simulink model "breaker_slower"  (R2023a)
settings: Solver=daessc  StartTime=0.0  StopTime=60*60*24  RelTol=1e-3
InitFcn:
  | to = 0.1;
  | V_G = 16.5e3;
  | V1 = 230e3;
  | V2 = 10.5e3;
  | V3 = 380;
  | 
  | P_G = 10e6;
  | S_T1 = 5e6;
  | S_T2 = S_T1;
undefined symbols (not defined in the file): A, B, C, D1, Dd, Delta, j
libraries: spsThreePhaseVIMeasurementLib x4, spsThreePhaseTransformerTwoWindingsLib x3, spsThreePhaseParallelRLCLoadLib x3, spsDistributedParametersLineLib x2, spsSeriesRLCBranchLib x2, spsControlledCurrentSourceLib x2, spsVoltageMeasurementLib x2, spsDieselMotorModel x1, spsExcitationSystemLib x1, spsPower3phPhasorLib x1, spsSynchronousMachinepuStandardLib x1, spsThreePhaseBreakerLib x1
settings Model: Creator=97033  LastModifiedBy=97033

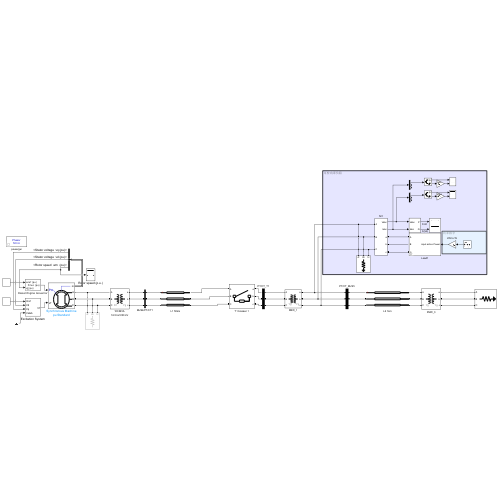
[thumbnail: Simulink's stored preview of the top-level diagram]
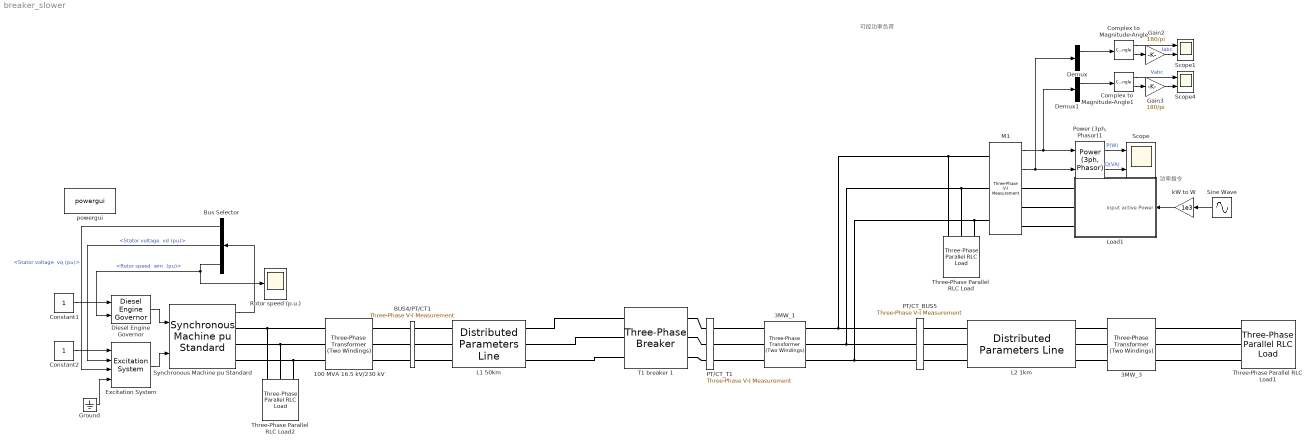
== system breaker_slower ==
  note: 功率指令
  note: 可控功率负荷
  100 MVA 16.5 kV/230 kV : spsThreePhaseTransformerTwoWindingsLib/Three-Phase Transformer (Two Windings)  Winding1Connection=Delta (D1)  Winding2Connection=Yg  CoreType=Three single-phase transformers  SetSaturation=off  Hysteresis=off  DataFile='hysteresis'  SetInitialFlux=off  Measurements=All measurements (V I Fluxes)  UNITS=pu  NominalPower=[P_G 50 ]  Winding1="[V_G 0.002  0.08]"  Winding2=[ V1 0.002 0.0576]  Rm=500  Lm=500  L0=0.5  Saturation="[ 0,0  ;  0.005,1.2  ;  1.0,1.4 ]"  InitialFluxes=[ 0.8 , -0.8 , 0.7 ]  BreakLoop=off  DiscreteSolver=Trapezoidal iterative  DataType=off  TransfoNumber=0
  3MW_1 : spsThreePhaseTransformerTwoWindingsLib/Three-Phase Transformer (Two Windings)  Winding1Connection=Yg  Winding2Connection=Yg  CoreType=Three single-phase transformers  SetSaturation=off  Hysteresis=off  DataFile='hysteresis'  SetInitialFlux=off  Measurements=None  UNITS=pu  NominalPower=[S_T1 , 50 ]  Winding1=[ V1 , 0.002 , 0.08 ]  Winding2=[ V2 , 0.002 , 0.08 ]  Rm=500  Lm=500  L0=0.5  Saturation=[ 0,0 ; 0.0024,1.2 ; 1.0,1.52 ]  InitialFluxes=[ 0.8 , -0.8 , 0.7 ]  BreakLoop=off  DiscreteSolver=Trapezoidal iterative  DataType=off  TransfoNumber=1
  3MW_3 : spsThreePhaseTransformerTwoWindingsLib/Three-Phase Transformer (Two Windings)  Winding1Connection=Yg  Winding2Connection=Yg  CoreType=Three single-phase transformers  SetSaturation=off  Hysteresis=off  DataFile='hysteresis'  SetInitialFlux=off  Measurements=None  UNITS=pu  NominalPower=[S_T1 , 50 ]  Winding1=[ V2 , 0.002 , 0.08 ]  Winding2=[ V3 , 0.002 , 0.08 ]  Rm=500  Lm=500  L0=0.5  Saturation=[ 0,0 ; 0.0024,1.2 ; 1.0,1.52 ]  InitialFluxes=[ 0.8 , -0.8 , 0.7 ]  BreakLoop=off  DiscreteSolver=Trapezoidal iterative  DataType=off  TransfoNumber=1
  BUS4/PT/CT1 : spsThreePhaseVIMeasurementLib/Three-Phase V-I Measurement  VoltageMeasurement=phase-to-ground  SetLabelV=on  LabelV=BUS4_Vabc  Vpu=off  VpuLL=off  CurrentMeasurement=yes  SetLabelI=on  LabelI=BUS4_Iabc  Ipu=off  Pbase=100e6  Vbase=500e3  OutputType=Complex  PhasorSimulation=on  PSBequivalent=0
  Bus Selector : BusSelector  OutputSignals="dq0 components.Stator voltage  vq (pu),dq0 components.Stator voltage  vd (pu),Mechanical.Rotor speed  wm  (pu)"
  Complex to Magnitude-Angle : ComplexToMagnitudeAngle
  Complex to Magnitude-Angle1 : ComplexToMagnitudeAngle
  Constant1 : Constant
  Constant2 : Constant
  Demux : Demux  Outputs=3
  Demux1 : Demux  Outputs=3
  Diesel Engine Governor : spsDieselMotorModel/Diesel Engine Governor  K=29  Tr=[0.01 0.02 0.2]  Ta=[0.25 0.009 0.0384]  Tlim=[0 1.1]  Td=0.024  Pm0=0.007343
  Excitation System : spsExcitationSystemLib/Excitation System  tr=20e-3  reg=[ 300, 0.001 ]  exc=[ 1, 0 ]  tgr=[ 0, 0 ]  damp=[ 0.001, 0.1 ]  sat=[ 0, 0 ]  lim=[ -11.5, 11.5, 0 ]  v0=[1 1.0072]
  Gain2 : Gain  Gain=180/pi
  Gain3 : Gain  Gain=180/pi
  Ground : Ground
  L1 50km : spsDistributedParametersLineLib/Distributed Parameters Line  Phases=3  Length=50  Frequency=50  Resistance="[0.1058  0.2758]"  Inductance="[2.3854e-3  3.220e-3]"  Capacitance="[17.65e-9  8.297e-9]"  x1=[8.11254497425638e-10 1435.76822832671 1413.84463935268;314.159265358979 314.159265358979 314.159265358979;-1.51704666570655 -1.26319034583497 -2.82717844992401]  x2=[7.80983845873745e-10 1443.20228947027 1421.37759574387;314.159265358979 314.159265358979 314.159265358979;-1.57738704185351 -1.26390237661045 -2.82798405384252]  x3=[3.89558894376792e-13 3.88420818677175 3.82284151982266;314.159265358979 314.159265358979 314.159265358979;-0.687252712637529 -1.36506185207182 -2.93068634651134]  x4=[2.29141256438702e-12 3.88291642642986 3.82686373555617;314.159265358979 314.159265358979 314.159265358979;-1.7204680603264 -1.26430606341361 -2.82682308359116]  x5=0.000324431464257091  V1=[1.093e-05 9.838e+04 9.838e+04;314.2 314.2 314.2;-0.3111 0.00854 -1.562]  V2=[1.093e-05 9.237e+04 9.237e+04;314.2 314.2 314.2;-0.3111 -0.2113 -1.782]  I1=[1.745e-08 2.849e+04 2.849e+04;314.2 314.2 314.2;-0.3423 2.9 1.329]  I2=[1.767e-08 2.9e+04 2.9e+04;314.2 314.2 314.2;-0.2816 -0.2391 -1.81]  nHarmo=1  Measurements=None  Decoupling=off  VsMag0=0  VrMag0=0  VsAngle0=0  VrAngle0=0  IsMag0=0  IrMag0=0  IsAngle0=0  IrAngle0=0
      settings: AttributesFormatString=\n
  L2 1km : spsDistributedParametersLineLib/Distributed Parameters Line  Phases=3  Length=1  Frequency=50  Resistance="[0.1058  0.2758]"  Inductance="[2.3854e-3  3.220e-3]"  Capacitance="[17.65e-9  8.297e-9]"  x1=[2.11924365740915e-09 78721.7359658811 223822.826299137;314.159265358979 314.159265358979 314.159265358979;-2.64962390305536 -0.00655028347033348 1.56395213727741]  x2=[2.12547837018316e-09 78715.0348375581 223803.77355008;314.159265358979 314.159265358979 314.159265358979;-2.64341726306893 -0.00667686374960178 1.56382555699814]  x3=[3.3655743288385e-11 199.928996109937 568.441135341219;314.159265358979 314.159265358979 314.159265358979;3.09267060703222 0.0270103950188096 1.59751281576664]  x4=[9.94540432532086e-12 228.454278999728 649.544649625245;314.159265358979 314.159265358979 314.159265358979;-1.5736701478916 -0.0379490943389389 1.53255332640882]  x5=6.48862928514182e-06  V1=[1.093e-05 9.838e+04 9.838e+04;314.2 314.2 314.2;-0.3111 0.00854 -1.562]  V2=[1.093e-05 9.237e+04 9.237e+04;314.2 314.2 314.2;-0.3111 -0.2113 -1.782]  I1=[1.745e-08 2.849e+04 2.849e+04;314.2 314.2 314.2;-0.3423 2.9 1.329]  I2=[1.767e-08 2.9e+04 2.9e+04;314.2 314.2 314.2;-0.2816 -0.2391 -1.81]  nHarmo=1  Measurements=None  Decoupling=off  VsMag0=0  VrMag0=0  VsAngle0=0  VrAngle0=0  IsMag0=0  IrMag0=0  IsAngle0=0  IrAngle0=0
      settings: AttributesFormatString=\n
  Load1 : Subsystem  mask{power_factor=1}
      mask DialogControl ParameterGroupVar Prompt: 参数
  M1 : spsThreePhaseVIMeasurementLib/Three-Phase V-I Measurement  VoltageMeasurement=phase-to-ground  SetLabelV=off  LabelV=V_Wind  Vpu=off  VpuLL=off  CurrentMeasurement=yes  SetLabelI=off  LabelI=I_Wind  Ipu=off  Pbase=6*1.5e6/0.9  Vbase=575  OutputType=Complex  PhasorSimulation=on  PSBequivalent=0
  PT/CT_BUS5 : spsThreePhaseVIMeasurementLib/Three-Phase V-I Measurement  VoltageMeasurement=phase-to-ground  SetLabelV=on  LabelV=BUS5_Vabc  Vpu=off  VpuLL=off  CurrentMeasurement=yes  SetLabelI=on  LabelI=BUS5_Iabc  Ipu=off  Pbase=6*1.5e6/0.9  Vbase=575  OutputType=Complex  PhasorSimulation=on  PSBequivalent=0
  PT/CT_T1 : spsThreePhaseVIMeasurementLib/Three-Phase V-I Measurement  VoltageMeasurement=phase-to-ground  SetLabelV=on  LabelV=V_T1  Vpu=off  VpuLL=off  CurrentMeasurement=yes  SetLabelI=on  LabelI=I_T1  Ipu=off  Pbase=6*1.5e6/0.9  Vbase=575  OutputType=Complex  PhasorSimulation=on  PSBequivalent=0
  "Power (3ph, Phasor)1" : spsPower3phPhasorLib/Power (3ph, Phasor)
  Rotor speed (p.u.) : Scope
  Scope : Scope  NumInputPorts=2
  Scope1 : Scope  NumInputPorts=2
  Scope4 : Scope  NumInputPorts=2
  Sine Wave : Sin  SineType=Sample based  Amplitude=5  Frequency=3600  SampleTime=60
  Synchronous Machine pu Standard : spsSynchronousMachinepuStandardLib/Synchronous Machine pu Standard  PresetModel=No  MechanicalLoad=Mechanical power Pm  ShowDetailedParameters=on  RotorType=Salient-pole  Units=per unit standard parameters  MeasurementBus=off  NominalParameters="[ P_G  V_G   50]"  Reactances1=[ 1.81, 0.3, 0.23, 1.76, 0.65, 0.25, 0.15 ]  Reactances2="[ 1.305, 0.296, 0.252, 0.474,  0.243,  0.18 ]"  dAxisTimeConstants=Open-circuit  qAxisTimeConstants=Short-circuit  TimeConstants1="[ 4.4849  0.0681  0.1  ]"  TimeConstants2=[ 8.0, 0.03, 1.0, 0.07 ]  TimeConstants3="[  4.49  0.0681  0.0513  ]"  TimeConstants4=[ 8.0, 0.03, 0.3371, 0.0295 ]  TimeConstants5=[ 1.01, 0.053, 0.1 ]  TimeConstants6=[ 1.3201, 0.023, 1.0, 0.07 ]  TimeConstants7=[0.012 0.003 0.003]  TimeConstants8=[ 1.3201, 0.0231, 0.3371, 0.0295 ]  StatorResistance=0.003  Mechanical=[3.7 0 1 ]  PolePairs=20  InitialConditions=[0 -89.802 0.00913935 0.00913935 0.00913935 -36.542 -156.542 83.458 1.00715]  SetSaturation=off  Saturation=[0.6404,0.7127,0.8441,0.9214,0.9956,1.082,1.19,1.316,1.457;0.7,0.7698,0.8872,0.9466,0.9969,1.046,1.1,1.151,1.201]  LoadFlowParameters=[1,0,0,0,0]  TsPowergui=0  TsBlock=-1  IterativeModel=Trapezoidal non iterative  IterativeDiscreteModel=Trapezoidal non iterative  BusType=swing  Pref=0  Qref=0  Qmin=-inf  Qmax=inf  PLF=0  QLF=0
  T1 breaker 1 : spsThreePhaseBreakerLib/Three-Phase Breaker  InitialState=open  SwitchA=on  SwitchB=on  SwitchC=on  SwitchTimes=0  External=off  BreakerResistance=1e-6  SnubberResistance=1e9  SnubberCapacitance=inf  Measurements=None
  Three-Phase Parallel RLC Load : spsThreePhaseParallelRLCLoadLib/Three-Phase Parallel RLC Load  LConnTagsString=A|B|C  Configuration=Y (grounded)  NominalVoltage=V2  Vabc=[1e3 1e3 1e3]  Vabcp=[1e3 1e3 1e3]  NominalFrequency=50  UnbalancedPower=off  ActivePower=1e6  InductivePower=0  CapacitivePower=0  Pabc=[10e3 9e3 11e3]  QLabc=[100 90 110]  QCabc=[100 90 110]  Pabcp=[10e3 9e3 11e3]  QLabcp=[100 90 110]  QCabcp=[100 90 110]  Measurements=None  LoadType=constant Z
  Three-Phase Parallel RLC Load1 : spsThreePhaseParallelRLCLoadLib/Three-Phase Parallel RLC Load  LConnTagsString=A|B|C  Configuration=Y (grounded)  NominalVoltage=V3  Vabc=[1e3 1e3 1e3]  Vabcp=[1e3 1e3 1e3]  NominalFrequency=50  UnbalancedPower=off  ActivePower=10e3  InductivePower=0  CapacitivePower=0  Pabc=[10e3 9e3 11e3]  QLabc=[100 90 110]  QCabc=[100 90 110]  Pabcp=[10e3 9e3 11e3]  QLabcp=[100 90 110]  QCabcp=[100 90 110]  Measurements=None  LoadType=constant Z
  Three-Phase Parallel RLC Load2 : spsThreePhaseParallelRLCLoadLib/Three-Phase Parallel RLC Load  LConnTagsString=A|B|C  Configuration=Y (floating)  NominalVoltage=V_G  Vabc=[1e3 1e3 1e3]  Vabcp=[1e3 1e3 1e3]  NominalFrequency=50  UnbalancedPower=off  ActivePower=1e3  InductivePower=0  CapacitivePower=0  Pabc=[10e3 9e3 11e3]  QLabc=[100 90 110]  QCabc=[100 90 110]  Pabcp=[10e3 9e3 11e3]  QLabcp=[100 90 110]  QCabcp=[100 90 110]  Measurements=None  LoadType=constant PQ
  kW to W : Gain  Gain=1e3
  powergui : sps_lib/powergui  Priority=1  SimulationMode=Phasor  SampleTime=50e-6  frequency=50  Iterations=50  frequencyindice=50  Pbase=100e6  ErrMax=1e-4  UnitsV=kV  UnitsW=MW  buscounter=0  FunctionMessages=off  echomessages=off  EnableUseOfTLC=off  CurrentSourceSwitches=off  DisableSnubberDevices=off  DisableRonSwitches=off  DisableVfSwitches=off  DisplayEquations=off  AutomaticDiscreteSolvers=off  SolverType=Tustin/Backward Euler (TBE)  Interpol=off  ExternalGateDelay=off  methode=off  Ts=100  x0status=blocks  SPID=on  SwTol=0  HookPort=off  NonlinearTolerance=1e-4  nMaxIteration=100  ContinueOnMaxIteration=off  RestoreLinks=warning  ResistiveCurrentMeasurement=off  Frange=[0:2:500]  Ylog=off  Xlog=on  ShowGrid=off  save=off  variable=ZData  structure=0  ZoomFFT=off  StartTime=0.0  cycles=1  DisplayStyle=1  fundamental=60  FreqAxis=off  MaxFrequency=1000  frequencyindicesteady=1  RmsSteady=1  display=off
  wires:
  Bus Selector/3 -> Diesel Engine Governor/2, Rotor speed (p.u.)/1  "<Rotor speed  wm  (pu)>"
  Ground/1 -> Excitation System/4
  Constant1/1 -> Diesel Engine Governor/1
  Bus Selector/1 -> Excitation System/3  "<Stator voltage  vq (pu)>"
  Constant2/1 -> Excitation System/1
  Diesel Engine Governor/1 -> Synchronous Machine pu Standard/1
  Bus Selector/2 -> Excitation System/2  "<Stator voltage  vd (pu)>"
  Excitation System/1 -> Synchronous Machine pu Standard/2
  Synchronous Machine pu Standard/1 -> Bus Selector/1
  Complex to Magnitude-Angle1/2 -> Gain3/1
  Complex to Magnitude-Angle1/1 -> Scope4/1  "Vabc"
  Complex to Magnitude-Angle/1 -> Scope1/1  "Iabc"
  Complex to Magnitude-Angle/2 -> Gain2/1
  Sine Wave/1 -> kW to W/1
  Demux1/1 -> Complex to Magnitude-Angle1/1
  Demux/1 -> Complex to Magnitude-Angle/1
  kW to W/1 -> Load1/1(input active Power)
  "Power (3ph, Phasor)1"/2 -> Scope/2  "Q(VA)"
  M1/2 -> Demux/1, "Power (3ph, Phasor)1"/2
  Gain3/1 -> Scope4/2
  Gain2/1 -> Scope1/2
  "Power (3ph, Phasor)1"/1 -> Scope/1  "P(W)"
  M1/1 -> Demux1/1, "Power (3ph, Phasor)1"/1
  connections:
  T1 breaker 1/LConn2 -- L1 50km/RConn2
  L1 50km/RConn1 -- T1 breaker 1/LConn1
  PT/CT_BUS5/RConn1 -- L2 1km/LConn1
  Three-Phase Parallel RLC Load2/LConn3 -- Synchronous Machine pu Standard/RConn3 -- 100 MVA 16.5 kV/230 kV/LConn3
  PT/CT_BUS5/RConn3 -- L2 1km/LConn3
  Synchronous Machine pu Standard/RConn2 -- Three-Phase Parallel RLC Load2/LConn2 -- 100 MVA 16.5 kV/230 kV/LConn2
  Three-Phase Parallel RLC Load/LConn1 -- 3MW_1/RConn1 -- PT/CT_BUS5/LConn1 -- M1/LConn1
  L1 50km/RConn3 -- T1 breaker 1/LConn3
  M1/LConn2 -- 3MW_1/RConn2 -- PT/CT_BUS5/LConn2 -- Three-Phase Parallel RLC Load/LConn2
  PT/CT_BUS5/RConn2 -- L2 1km/LConn2
  M1/LConn3 -- 3MW_1/RConn3 -- PT/CT_BUS5/LConn3 -- Three-Phase Parallel RLC Load/LConn3
  Synchronous Machine pu Standard/RConn1 -- Three-Phase Parallel RLC Load2/LConn1 -- 100 MVA 16.5 kV/230 kV/LConn1
  3MW_3/RConn2 -- Three-Phase Parallel RLC Load1/LConn2
  PT/CT_T1/RConn1 -- 3MW_1/LConn1
  3MW_3/LConn3 -- L2 1km/RConn3
  3MW_3/LConn1 -- L2 1km/RConn1
  L1 50km/LConn2 -- BUS4/PT/CT1/RConn2
  BUS4/PT/CT1/LConn2 -- 100 MVA 16.5 kV/230 kV/RConn2
  L1 50km/LConn3 -- BUS4/PT/CT1/RConn3
  PT/CT_T1/RConn2 -- 3MW_1/LConn2
  L1 50km/LConn1 -- BUS4/PT/CT1/RConn1
  Three-Phase Parallel RLC Load1/LConn1 -- 3MW_3/RConn1
  BUS4/PT/CT1/LConn1 -- 100 MVA 16.5 kV/230 kV/RConn1
  T1 breaker 1/RConn3 -- PT/CT_T1/LConn3
  3MW_3/LConn2 -- L2 1km/RConn2
  PT/CT_T1/RConn3 -- 3MW_1/LConn3
  BUS4/PT/CT1/LConn3 -- 100 MVA 16.5 kV/230 kV/RConn3
  T1 breaker 1/RConn1 -- PT/CT_T1/LConn1
  T1 breaker 1/RConn2 -- PT/CT_T1/LConn2
  Three-Phase Parallel RLC Load1/LConn3 -- 3MW_3/RConn3
  Load1/RConn2 -- M1/RConn2
  Load1/RConn3 -- M1/RConn3
  Load1/RConn1 -- M1/RConn1

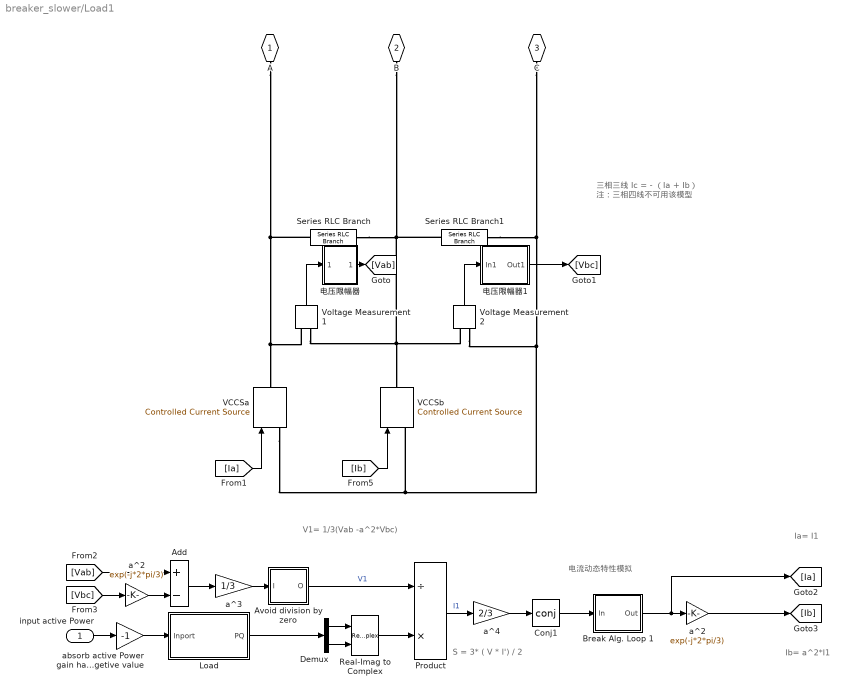
== system breaker_slower/Load1 ==
  note: 三相三线 Ic = - （Ia + Ib）
      | 注：三相四线不可用该模型
  note: 电流动态特性模拟
  note: Ia= I1
  note: V1= 1/3(Vab -a^2*Vbc)
  note: Ib= a^2*I1
  note: S = 3* ( V * I') / 2
  input active Power : Inport
  Add : Sum  Inputs=+-
  Avoid division by zero : Subsystem
  Break Alg. Loop 1 : Subsystem
  Conj1 : Math  Operator=conj  SignedPower=on
  Demux : Demux  Outputs=2
  Load : Subsystem
  Product : Product  Inputs=/*  InputSameDT=on  SaturateOnIntegerOverflow=on  OutDataTypeStr=Inherit: Same as first input
  Real-Imag to Complex : RealImagToComplex
  Series RLC Branch : spsSeriesRLCBranchLib/Series RLC Branch  LConnTagsString=__new0  RConnTagsString=__new0  BranchType=R  Resistance=1e6  Inductance=1e-3  SetiL0=off  InitialCurrent=0  Capacitance=1e-6  Setx0=off  InitialVoltage=0  Measurements=None
  Series RLC Branch1 : spsSeriesRLCBranchLib/Series RLC Branch  LConnTagsString=__new0  RConnTagsString=__new0  BranchType=R  Resistance=1e6  Inductance=1e-3  SetiL0=off  InitialCurrent=0  Capacitance=1e-6  Setx0=off  InitialVoltage=0  Measurements=None
  VCCSa : spsControlledCurrentSourceLib/Controlled Current Source  Initialize=on  Source_Type=AC  Amplitude=1000  Phase=180/pi  Frequency=50  Measurements=Current
  VCCSb : spsControlledCurrentSourceLib/Controlled Current Source  Initialize=on  Source_Type=AC  Amplitude=1000  Phase=(2*pi/3)*180/pi  Frequency=50  Measurements=Current
  Voltage Measurement1 : spsVoltageMeasurementLib/Voltage Measurement  PhasorSimulation=on  OutputType=Complex  PSBequivalent=0
  Voltage Measurement2 : spsVoltageMeasurementLib/Voltage Measurement  PhasorSimulation=on  OutputType=Complex  PSBequivalent=0
  a^2 : Gain  Gain=exp(-j*2*pi/3)  SaturateOnIntegerOverflow=on  OutDataTypeStr=Inherit: Same as input  ParamDataTypeStr=Inherit: Same as input
  "a^2 " : Gain  Gain=exp(-j*2*pi/3)  SaturateOnIntegerOverflow=on  OutDataTypeStr=Inherit: Same as input  ParamDataTypeStr=Inherit: Same as input
  a^3 : Gain  Gain=1/3  SaturateOnIntegerOverflow=on  OutDataTypeStr=Inherit: Same as input  ParamDataTypeStr=Inherit: Same as input
  a^4 : Gain  Gain=2/3  SaturateOnIntegerOverflow=on  OutDataTypeStr=Inherit: Same as input  ParamDataTypeStr=Inherit: Same as input
  absorb active Power gain has a nagetive value : Gain  Gain=-1
  电压限幅器 : Subsystem
  电压限幅器1 : Subsystem
  A : PMIOPort  Tag=PMCPort  Side=Right
  B : PMIOPort  Tag=PMCPort  Port=2  Side=Right
  C : PMIOPort  Tag=PMCPort  Port=3  Side=Right
  wires:
  a^3/1 -> Avoid division by zero/1(I)
  [Vab] -> Add/1
  [Ia] -> VCCSa/1
  Avoid division by zero/1(O) -> Product/1  "V1"
  [Vbc] -> "a^2 "/1
  absorb active Power gain has a nagetive value/1 -> Load/1(Inport)
  "a^2 "/1 -> Add/2
  Real-Imag to Complex/1 -> Product/2
  [Ib] -> VCCSb/1
  Product/1 -> a^4/1  "I1"
  Add/1 -> a^3/1
  a^4/1 -> Conj1/1
  Demux/1 -> Real-Imag to Complex/1
  input active Power/1 -> absorb active Power gain has a nagetive value/1
  Demux/2 -> Real-Imag to Complex/2
  Break Alg. Loop 1/1(Out) -> [Ia], a^2/1
  Conj1/1 -> Break Alg. Loop 1/1(In)
  a^2/1 -> [Ib]
  Load/1(PQ) -> Demux/1
  Voltage Measurement1/1 -> 电压限幅器/1(In1)
  电压限幅器/1(Out1) -> [Vab]
  Voltage Measurement2/1 -> 电压限幅器1/1(In1)
  电压限幅器1/1(Out1) -> [Vbc]
  connections:
  Voltage Measurement1/LConn1 -- A/RConn1 -- Series RLC Branch/LConn1 -- VCCSa/RConn1
  Series RLC Branch1/RConn1 -- C/RConn1 -- Voltage Measurement2/LConn2 -- VCCSa/LConn1 -- VCCSb/LConn1
  Series RLC Branch/RConn1 -- B/RConn1 -- Series RLC Branch1/LConn1 -- Voltage Measurement1/LConn2 -- VCCSb/RConn1 -- Voltage Measurement2/LConn1

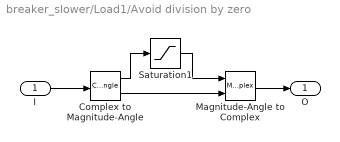
== system breaker_slower/Load1/Avoid division by zero ==
  I : Inport
  Complex to Magnitude-Angle : ComplexToMagnitudeAngle
  Magnitude-Angle to Complex : MagnitudeAngleToComplex
  Saturation1 : Saturate  UpperLimit=inf  LowerLimit=1e-6
  O : Outport  VectorParamsAs1DForOutWhenUnconnected=off
  wires:
  I/1 -> Complex to Magnitude-Angle/1
  Saturation1/1 -> Magnitude-Angle to Complex/1
  Complex to Magnitude-Angle/1 -> Saturation1/1
  Magnitude-Angle to Complex/1 -> O/1
  Complex to Magnitude-Angle/2 -> Magnitude-Angle to Complex/2

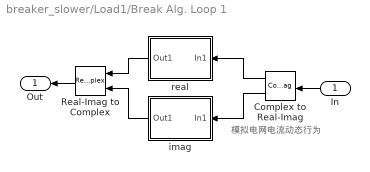
== system breaker_slower/Load1/Break Alg. Loop 1 ==
  note: 模拟电网电流动态行为
  In : Inport
  Complex to Real-Imag : ComplexToRealImag
  Real-Imag to Complex : RealImagToComplex
  imag : Subsystem  mask(Transfer Function with Initial Outputs){N=[1], D=[0.1  1], Y0=0, U0=0}
      mask prompts: N "Numerator:"; D "Denominator:"; Y0 "Initial output:"; U0 "Initial input:"
      mask help: Vector expressions for numerator, and denominator. Coefficients are in descending powers of s.
      mask init:
      | [A,B,C,Dd]=tf2ss(N,D);if (isempty(Y0));[m,n]=size(A);X0=zeros(1,m); end; if (isempty(U0));[m,p]=size(B);U0=zeros(1,p);end;X0=getxo(A,B,C,Dd,U0,Y0,0);
      mask Help: Specify the initial output for the transfer function.  An optimization routine attempts to determine the appropriate initial states so that the specified initial output is achieved.  For more details, see the m-file getxo.m
      mask Display: dpoly(N,D,'s')
  real : Subsystem  mask(Transfer Function with Initial Outputs){N=[1], D=[0.1 1], Y0=0, U0=0}
      mask prompts: N "Numerator:"; D "Denominator:"; Y0 "Initial output:"; U0 "Initial input:"
      mask help: Vector expressions for numerator, and denominator. Coefficients are in descending powers of s.
      mask init:
      | [A,B,C,Dd]=tf2ss(N,D);if (isempty(Y0));[m,n]=size(A);X0=zeros(1,m); end; if (isempty(U0));[m,p]=size(B);U0=zeros(1,p);end;X0=getxo(A,B,C,Dd,U0,Y0,0);
      mask Help: Specify the initial output for the transfer function.  An optimization routine attempts to determine the appropriate initial states so that the specified initial output is achieved.  For more details, see the m-file getxo.m
      mask Display: dpoly(N,D,'s')
  Out : Outport  VectorParamsAs1DForOutWhenUnconnected=off
  wires:
  Complex to Real-Imag/1 -> real/1(In1)
  Complex to Real-Imag/2 -> imag/1(In1)
  In/1 -> Complex to Real-Imag/1
  Real-Imag to Complex/1 -> Out/1
  real/1(Out1) -> Real-Imag to Complex/1
  imag/1(Out1) -> Real-Imag to Complex/2

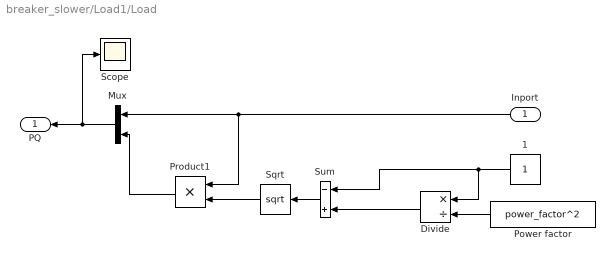
== system breaker_slower/Load1/Load ==
  Inport : Inport
  1 : Constant
  Divide : Product  Inputs=*/
  Mux : Mux  Inputs=2
  Power factor : Constant  Value=power_factor^2
  Product1 : Product
  Scope : Scope
  Sqrt : Sqrt
  Sum : Sum  Inputs=-+
  PQ : Outport  VectorParamsAs1DForOutWhenUnconnected=off
  wires:
  Inport/1 -> Product1/1, Mux/1
  Mux/1 -> Scope/1, PQ/1
  Sqrt/1 -> Product1/2
  Product1/1 -> Mux/2
  Divide/1 -> Sum/2
  1/1 -> Sum/1, Divide/1
  Power factor/1 -> Divide/2
  Sum/1 -> Sqrt/1

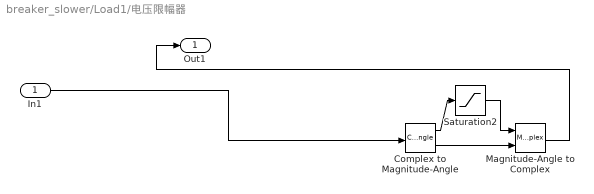
== system breaker_slower/Load1/电压限幅器 ==
  In1 : Inport
  Complex to Magnitude-Angle : ComplexToMagnitudeAngle
  Magnitude-Angle to Complex : MagnitudeAngleToComplex
  Saturation2 : Saturate  UpperLimit=50e3  LowerLimit=-50e3
  Out1 : Outport
  wires:
  Saturation2/1 -> Magnitude-Angle to Complex/1
  Complex to Magnitude-Angle/2 -> Magnitude-Angle to Complex/2
  In1/1 -> Complex to Magnitude-Angle/1
  Magnitude-Angle to Complex/1 -> Out1/1
  Complex to Magnitude-Angle/1 -> Saturation2/1

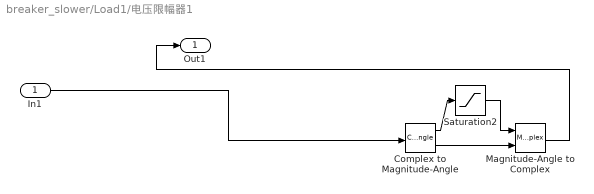
== system breaker_slower/Load1/电压限幅器1 ==
  In1 : Inport
  Complex to Magnitude-Angle : ComplexToMagnitudeAngle
  Magnitude-Angle to Complex : MagnitudeAngleToComplex
  Saturation2 : Saturate  UpperLimit=50e3  LowerLimit=-50e3
  Out1 : Outport
  wires:
  Complex to Magnitude-Angle/1 -> Saturation2/1
  Magnitude-Angle to Complex/1 -> Out1/1
  In1/1 -> Complex to Magnitude-Angle/1
  Complex to Magnitude-Angle/2 -> Magnitude-Angle to Complex/2
  Saturation2/1 -> Magnitude-Angle to Complex/1

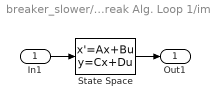
== system breaker_slower/Load1/Break Alg. Loop 1/imag ==
  In1 : Inport
  State Space : StateSpace  A=A  B=B  C=C  D=Dd  InitialCondition=X0
  Out1 : Outport  InitialOutput=0  VectorParamsAs1DForOutWhenUnconnected=off
  wires:
  State Space/1 -> Out1/1
  In1/1 -> State Space/1

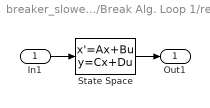
== system breaker_slower/Load1/Break Alg. Loop 1/real ==
  In1 : Inport
  State Space : StateSpace  A=A  B=B  C=C  D=Dd  InitialCondition=X0
  Out1 : Outport  InitialOutput=0  VectorParamsAs1DForOutWhenUnconnected=off
  wires:
  State Space/1 -> Out1/1
  In1/1 -> State Space/1
